simulink model "QModel"  (Simulink 8.4)
settings: Solver=ode45  StartTime=0.0  StopTime=20.0  RelTol=1e-3
undefined symbols (not defined in the file or in its folder): gain, initialCondition, par, regval
settings Model: Creator=marilena  LastModifiedBy=marilena
settings DebuggingCC: FcnCallInpInsideContextMsg=EnableAllAsWarning
settings GRTTargetCC: CombineOutputUpdateFcns=on  GRTInterface=off

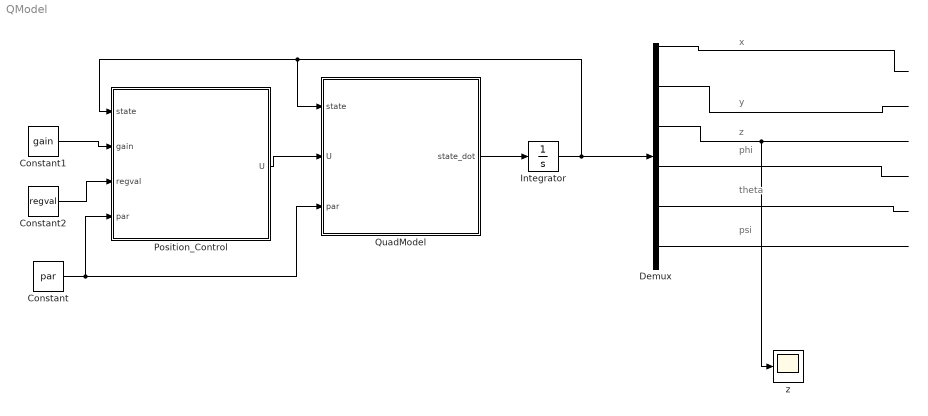
== system QModel ==
  note: x
  note: y
  note: z
  note: phi
  note: theta
  note: psi
  Constant : Constant  Value=par
  Constant1 : Constant  Value=gain
  Constant2 : Constant  Value=regval
  Demux : Demux  Outputs=12
  Integrator : Integrator  InitialCondition=initialCondition
  "Position_Control " : MATLAB Function  TreatAsAtomicUnit=on
  QuadModel : MATLAB Function  TreatAsAtomicUnit=on
  z : Scope
  wires:
  Demux/1 -> ?
  Demux/3 -> ?
  Demux/5 -> z/1
  Demux/7 -> ?
  Demux/9 -> ?
  Demux/11 -> ?
  QuadModel/1(state_dot) -> Integrator/1
  "Position_Control "/1(U) -> QuadModel/2(U)
  Constant2/1 -> "Position_Control "/3(regval)
  Constant1/1 -> "Position_Control "/2(gain)
  Integrator/1 -> QuadModel/1(state), "Position_Control "/1(state), Demux/1
  Constant/1 -> QuadModel/3(par), "Position_Control "/4(par)

== matlab function Position_Control  ==
  data: state input double; U output double; gain input double; regval input double; par input double
function U = Height_Control(state,gain,regval,par)

%model parameters
m=par(1);
m1=par(2);
Ix=par(3);
Iy=par(4);
Iz=par(5);
Ir=par(6);
Om_r=par(7);
d=par(8);
l=par(9);
g=par(10);

%controller gains
kx=gain(1);
kx_d=gain(2);
kx_i=gain(3);

ky=gain(4);
ky_d=gain(5);
ky_i=gain(6);

kz=gain(7);
kz_d=gain(8);
kz_i=gain(9);

k_phi=gain(10);
kphi_d=gain(11);
kphi_i=gain(12);

k_theta=gain(13);
ktheta_d=gain(14);
ktheta_i=gain(15);

k_psi=gain(16);
kpsi_d=gain(17);
kpsi_i=gain(18);

%regulation values
x_d=regval(1);
y_d=regval(2);
z_d=regval(3);
phi_d=regval(4);
theta_d=regval(5);
psi_d=regval(6);

%position
x=state(1);
vx=state(2);
y=state(3);
vy=state(4);
z=state(5);
vz=state(6);

%attitude
phi=state(7);
dphi=state(8);
theta=state(9);
dtheta=state(10);
psi=state(11);
dpsi=state(12);

% height control (U1=thrust)
stab_z=(g + kz*(z_d -z) + kz_d*(-vz));
fl_z=(m/(cos(phi)*cos(theta)));
U1=fl_z*stab_z;

U2=Ix*(k_phi * (phi_d - phi) + kphi_d * (-dphi));
U3=Iy*(k_theta * (theta_d - theta) + ktheta_d * (-dtheta));
U4=Iz*(k_psi * (psi_d - psi) + kpsi_d * (-dpsi));

U = [U1, U2, U3, U4]';

== matlab function QuadModel ==
  data: state input double; U input double; state_dot output double; par input double
function state_dot = quadrotor_model(state,U,par)

%model parameters
m=par(1);
m1=par(2);
Ix=par(3);
Iy=par(4);
Iz=par(5);
Ir=par(6);
Om_r=par(7);
d=par(8);
l=par(9);
g=par(10);

%position
x=state(1);
vx=state(2);
y=state(3);
vy=state(4);
z=state(5);
vz=state(6);

%attitude
phi=state(7);
dphi=state(8);
theta=state(9);
dtheta=state(10);
psi=state(11);
dpsi=state(12);

%control
U1=U(1);
U2=U(2);
U3=U(3);
U4=U(4);

%dynamics
xdot=vx;
vxdot = (U1/m)*(cos(phi)*sin(theta)*cos(psi)+sin(phi)*sin(psi));

ydot=vy;
vydot = (U1/m)*(cos(phi)*sin(theta)*sin(psi)-sin(phi)*cos(psi));

zdot=vz;
vzdot = - g + (U1/m)*(cos(phi)*cos(theta));

phidot=dphi;
dphidot =  ((Iy-Iz)/Ix)*dtheta*dpsi + (Ir/Ix)*dtheta*Om_r +(l/Ix)*U2; %;

thetadot=dtheta;
dthetadot = ((Iz-Ix)/Iy)*dphi*dpsi - (Ir/Iy)*dphi*Om_r +(l/Iy)*U3;  %;

psidot=dpsi;
dpsidot =  ((Ix-Iy)/Iz)*dphi*dtheta + (1/Iz)*U4; %;

state_dot = [xdot, vxdot, ydot, vydot, zdot, vzdot, phidot, dphidot, thetadot, dthetadot, psidot, dpsidot]';
